simulink model "g729_encoder_test"  (Simulink 8.1)
settings: Solver=ode45  StartTime=0.0  StopTime=100000  RelTol=1e-3
libraries: xbsIndex_r4 x17
settings Model: Creator=aruls  LastModifiedBy=aruls
settings DataIOCC: SignalLoggingSaveFormat=Dataset
settings OptimizationCC: ExpressionDepthLimit=128
settings DebuggingCC: FcnCallInpInsideContextMsg=EnableAllAsError
settings GRTTargetCC: CombineOutputUpdateFcns=on  GRTInterface=off

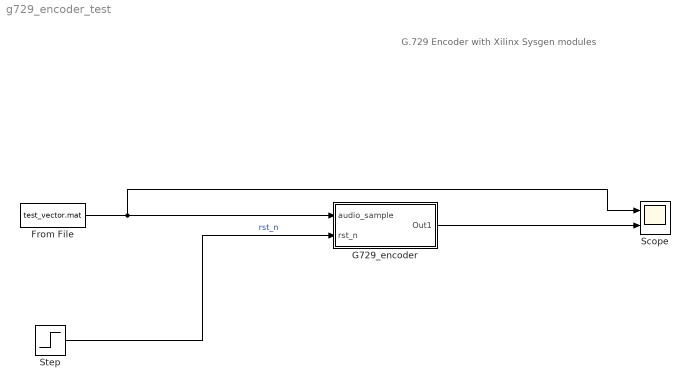
== system g729_encoder_test ==
  note: G.729 Encoder with Xilinx Sysgen modules
  From File : FromFile  FileName=test_vector.mat  SampleTime=1000
  G729_encoder : Subsystem
  Scope : Scope  NumInputPorts=2
      settings: YMin=-5~-5  YMax=5~5
  Step : Step  SampleTime=1000
  wires:
  From File/1 -> G729_encoder/1(audio_sample), Scope/1
  G729_encoder/1(Out1) -> Scope/2
  Step/1 -> G729_encoder/2(rst_n)  "rst_n"

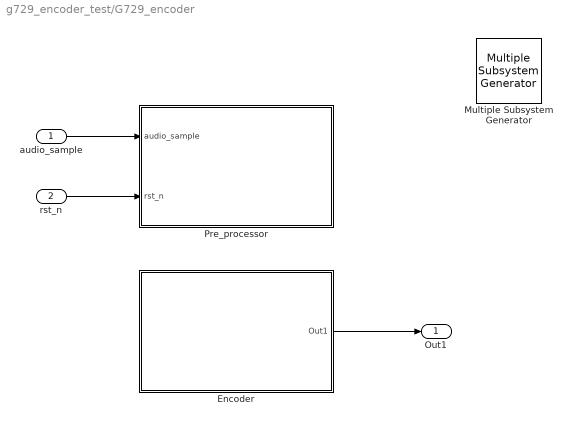
== system g729_encoder_test/G729_encoder ==
  audio_sample : Inport
  rst_n : Inport  Port=2
  Encoder : Subsystem
  Multiple Subsystem Generator : xbsIndex_r4/Multiple Subsystem Generator  Tag=xlStitcher  block_type=multiple_subsystem_generator
      settings: infoedit=Multiple Subsystem\nGenerator
  Pre_processor : Subsystem
  Out1 : Outport
  wires:
  audio_sample/1 -> Pre_processor/1(audio_sample)
  rst_n/1 -> Pre_processor/2(rst_n)
  Encoder/1(Out1) -> Out1/1

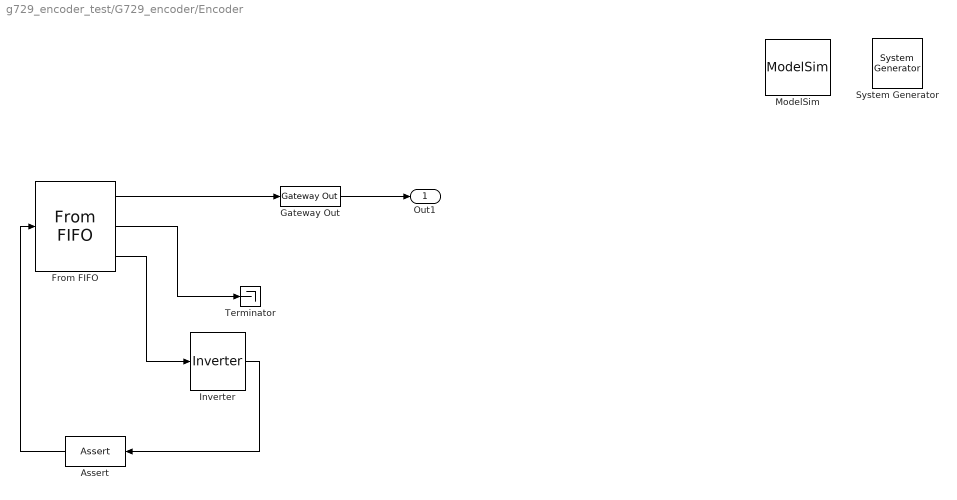
== system g729_encoder_test/G729_encoder/Encoder ==
  " System Generator" : xbsIndex_r4/ System Generator  Tag=genX  xilinxfamily=kintex7  part=xc7k325t  speed=-3  package=fbg676  synthesis_tool=XST  clock_wrapper=Clock Enables  directory=./netlist  proj_type=Project Navigator  Synth_file=XST Defaults  Impl_file=ISE Defaults  testbench=off  simulink_period=1  sysclk_period=15.625  dcm_input_clock_period=10  incr_netlist=off  trim_vbits=Everywhere in SubSystem  dbl_ovrd=According to Block Masks  core_generation=According to Block Masks  run_coregen=off  deprecated_control=off  eval_field=0  block_type=sysgen
  Assert : xbsIndex_r4/Assert  assert_type=on  type_source=Explicitly  gui_display_data_type=Boolean  arith_type=Boolean  n_bits=16  bin_pt=14  preci_type=Single  exp_width=8  frac_width=24  assert_rate=off  rate_source=Explicitly  period=1  output_port=on  block_type=assert
  From FIFO : xbsIndex_r4/From FIFO  shared_memory_name='audio_sample_fifo'  ownership=Owned elsewhere  mem_type=Block RAM  performance_options=Standard_FIFO  infoedit1=Available only for V4, V5, V6, V7, K7, A7 and Zynq devices.  embedded_registers=off  depth=512K  percent_nbits=4  has_arst=off  use_percent_full_port=on  gui_display_data_type=Fixed-point  arith_type="Signed  (2's comp)"  n_bits=16  bin_pt=14  preci_type=Single  dbl_ovrd=off  block_type=fromfifo
      settings: AttributesFormatString=<< %<shared_memory_name> >>  infoedit=First-in-first-out (FIFO) block that reads FIFO data from shared memory storage.
  Gateway Out : xbsIndex_r4/Gateway Out  inherit_from_input=off  hdl_port=on  timing_constraint=None  locs_specified=off  LOCs={}  UseAsDAC=off  DACChannel='1'  block_type=gatewayout
  Inverter : xbsIndex_r4/Inverter  en=off  latency=0  dbl_ovrd=off  block_type=inv
  ModelSim : xbsIndex_r4/ModelSim  dir=./modelsim  waveform=on  leave_open=on  skip_compile=off  use_unisim=off  use_ver_xilinxcorelib=off  custom_scripts=off  startup_timeout=40  block_type=hdlcosim
      settings: infoedit="Allow other blocks to schedule HDL co-simulation tasks.<br><br>Note that selecting \"Skip compilation\" when inappropriate can cause simulation errors and failures. Please refer to the block help for details."
  Terminator : Terminator
  Out1 : Outport
  wires:
  From FIFO/1 -> Gateway Out/1
  Gateway Out/1 -> Out1/1
  From FIFO/2 -> Terminator/1
  From FIFO/3 -> Inverter/1
  Inverter/1 -> Assert/1
  Assert/1 -> From FIFO/1

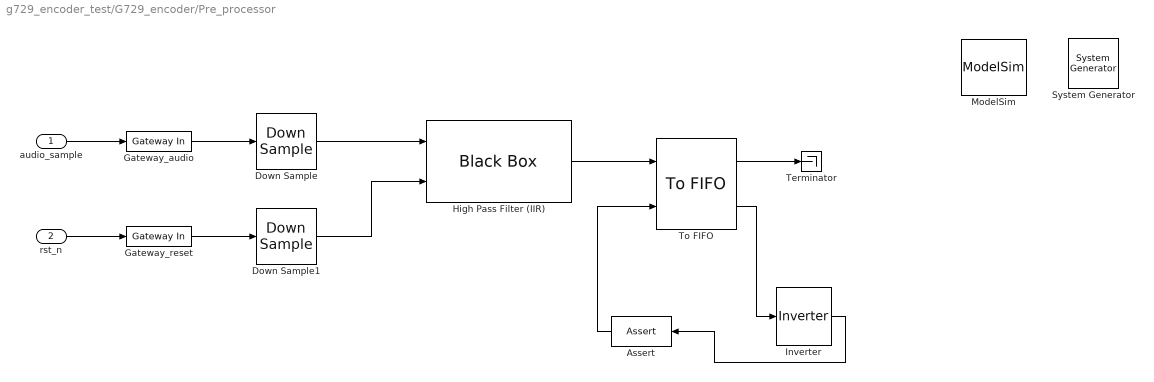
== system g729_encoder_test/G729_encoder/Pre_processor ==
  audio_sample : Inport
  rst_n : Inport  Port=2
  " System Generator" : xbsIndex_r4/ System Generator  Tag=genX  xilinxfamily=kintex7  part=xc7k325t  speed=-3  package=fbg676  synthesis_tool=XST  clock_wrapper=Clock Enables  directory=./netlist  proj_type=Project Navigator  Synth_file=XST Defaults  Impl_file=ISE Defaults  testbench=off  simulink_period=1  sysclk_period=15.625  dcm_input_clock_period=10  incr_netlist=off  trim_vbits=Everywhere in SubSystem  dbl_ovrd=According to Block Masks  core_generation=According to Block Masks  run_coregen=off  deprecated_control=off  eval_field=0  block_type=sysgen
  Assert : xbsIndex_r4/Assert  assert_type=off  type_source=Explicitly  gui_display_data_type=Fixed-point  arith_type="Signed  (2's comp)"  n_bits=16  bin_pt=14  preci_type=Single  exp_width=8  frac_width=24  assert_rate=off  rate_source=Explicitly  period=1  output_port=on  block_type=assert
  Down Sample : xbsIndex_r4/Down Sample  sample_ratio=2000  sample_phase="Last Value of Frame  (most efficient)"  en=off  latency=1  dbl_ovrd=off  block_type=dsamp
  Down Sample1 : xbsIndex_r4/Down Sample  sample_ratio=2000  sample_phase="Last Value of Frame  (most efficient)"  en=off  latency=1  dbl_ovrd=off  block_type=dsamp
  Gateway_audio : xbsIndex_r4/Gateway In  gui_display_data_type=Fixed-point  arith_type="Signed  (2's comp)"  n_bits=16  bin_pt=14  preci_type=Single  exp_width=8  frac_width=24  quantization="Round  (unbiased: +/- Inf)"  overflow=Saturate  period=1  dbl_ovrd=off  timing_constraint=None  locs_specified=off  LOCs={}  UseAsADC=off  ADCChannel='1'  inherit_from_input=off  hdl_port=on  block_type=gatewayin
  Gateway_reset : xbsIndex_r4/Gateway In  gui_display_data_type=Boolean  arith_type=Boolean  n_bits=16  bin_pt=14  preci_type=Single  exp_width=8  frac_width=24  quantization="Round  (unbiased: +/- Inf)"  overflow=Saturate  period=1  dbl_ovrd=off  timing_constraint=None  locs_specified=off  LOCs={}  UseAsADC=off  ADCChannel='1'  inherit_from_input=off  hdl_port=on  block_type=gatewayin
  High Pass Filter (IIR) : xbsIndex_r4/Black Box  init_code=high_pass_filter_config  sim_method=External co-simulator  engine_block=ModelSim  verbose=off  block_type=blackbox2
  Inverter : xbsIndex_r4/Inverter  en=off  latency=0  dbl_ovrd=off  block_type=inv
  ModelSim : xbsIndex_r4/ModelSim  dir=./modelsim  waveform=on  leave_open=on  skip_compile=off  use_unisim=off  use_ver_xilinxcorelib=off  custom_scripts=off  startup_timeout=40  block_type=hdlcosim
      settings: infoedit="Allow other blocks to schedule HDL co-simulation tasks.<br><br>Note that selecting \"Skip compilation\" when inappropriate can cause simulation errors and failures. Please refer to the block help for details."
  Terminator : Terminator
  To FIFO : xbsIndex_r4/To FIFO  shared_memory_name='audio_sample_fifo'  ownership=Locally owned  mem_type=Block RAM  performance_options=Standard_FIFO  infoedit1=Available only for V4, V5, V6, V7, K7, A7 and Zynq devices.  embedded_registers=off  depth=512K  percent_nbits=5  has_arst=off  use_percent_full_port=on  explicit_data_type=off  gui_display_data_type=Fixed-point  arith_type="Signed  (2's comp)"  n_bits=16  bin_pt=14  preci_type=Single  dbl_ovrd=off  block_type=tofifo
      settings: AttributesFormatString=<< %<shared_memory_name> >>  infoedit=First-in-first-out (FIFO) block that writes FIFO data to shared memory storage.
  wires:
  audio_sample/1 -> Gateway_audio/1
  Gateway_audio/1 -> Down Sample/1
  Down Sample/1 -> High Pass Filter (IIR)/1
  Down Sample1/1 -> High Pass Filter (IIR)/2
  High Pass Filter (IIR)/1 -> To FIFO/1
  To FIFO/1 -> Terminator/1
  rst_n/1 -> Gateway_reset/1
  Gateway_reset/1 -> Down Sample1/1
  To FIFO/2 -> Inverter/1
  Inverter/1 -> Assert/1
  Assert/1 -> To FIFO/2
